simulink model "BatterySimulation"  (R2024a)
settings: Solver=VariableStepAuto  StartTime=0.0  StopTime=inf  FixedStep=minStep  MaxStep=(1e-5)*1000  MinStep=1e-5  RelTol=1e-3
libraries: fl_lib x7, nesl_utility x4, batteryecm_lib x1, simulink x1
settings Model: SimulationMode=accelerator  Creator=nsu  LastModifiedBy=nsu

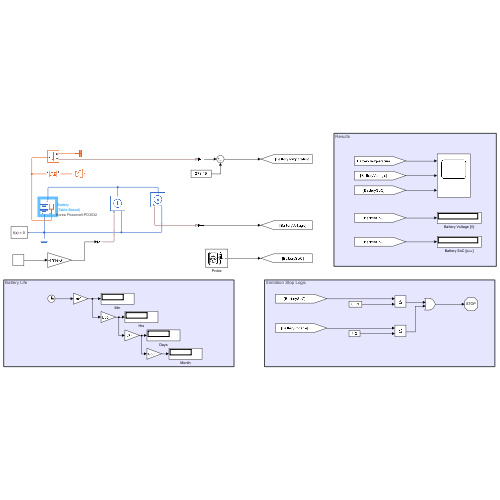
[thumbnail: Simulink's stored preview of the top-level diagram]
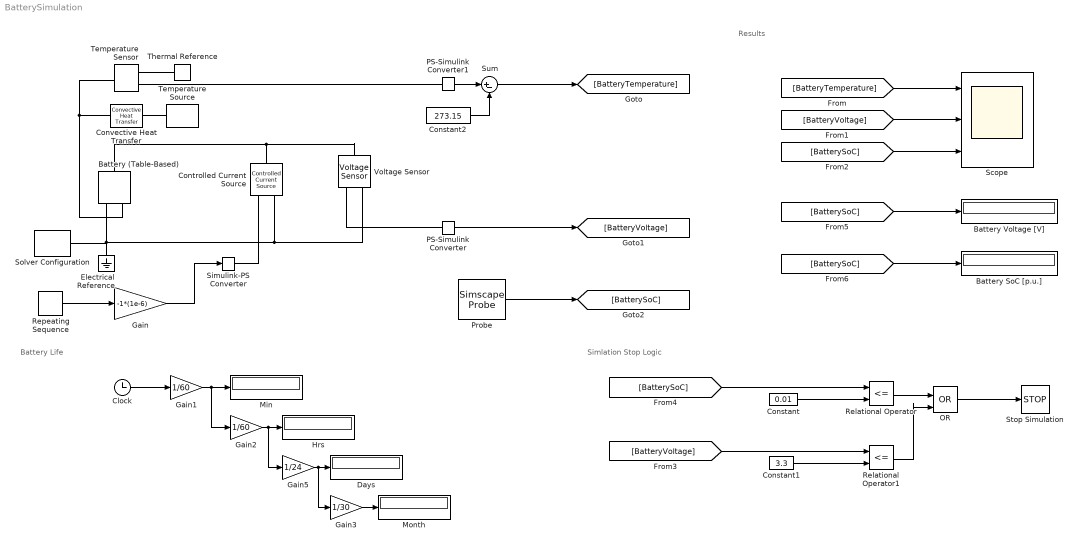
== system BatterySimulation ==
  note: Results
  note: Simlation Stop Logic
  note: Battery Life
  Battery (Table-Based) : batteryecm_lib/Battery (Table-Based)  Tag={'toolbox/physmod/battery/shared_library/m/batteryecm_lib_parts';'Battery__Table_Based_/Korea_Powercell/PD3032.xml'}  SOC_vec=[0 0.01 0.02 0.03 0.04 0.05 0.06 0.07 0.08 0.09 0.1 0.11 0.12 0.13 0.14 0.15 0.16 0.17 0.18 0.19 0.2 0.21 0.22 0.23 0.24 0.25 0.26 0.27 0.28 0.29 0.3 0.31 0.32 0.33 0.34 0.35 0.36 0.37 0.38 0.39 0.4 0.41 0.42 0.43 0.44 0.45 0.46 0.47 0.48 0.49 0.5 0.51 0.52 0.53 0.54 0.55 0.56 0.57 0.58 0.59 0.6 0.61 0.62 0.63 0.64 0.65 0.66 0.67 0.68 0.69 0.7 0.71 0.72 0.73 0.74 0.75 0.76 0.77 0.78 0.79 0.8 0.81 0.82 0.83 0.84 0.85 0.86 0.87 0.88 0.89 0.9 0.91 0.92 0.93 0.94 0.95 0.96 0.97 0.98 0.99 1]  T_dependence=simscape.enum.tablebattery.temperature_dependence.yes  prm_dir=simscape.enum.tablebattery.prm_dir.noCurrentDirectionality  T_vec=[-20 -10 25] degC  V0_mat=[2.95724 2.95724 2.95724;3.3564 3.3564 3.3564;3.49366 3.49366 3.49366;3.58258 3.58258 3.58258;3.63766 3.63766 3.63766;3.68332 3.68332 3.68332;3.70873 3.70873 3.70873;3.73055 3.73055 3.73055;3.74166 3.74166 3.74166;3.74045 3.74045 3.74045;3.73776 3.73776 3.73776;3.73631 3.73631 3.73631;3.73521 3.73521 3.73521;3.73661 3.73661 3.73661;3.73787 3.73787 3.73787;3.73862 3.73862 3.73862;3.74076 3.74076 3.74076;3.74303 3.74303 3.74303;3.74502 3.74502 3.74502;3.7472 3.7472 3.7472;3.74981 3.74981 3.74981;3.75229 3.75229 3.75229;3.7538 3.7538 3.7538;3.75584 3.75584 3.75584;3.75779 3.75779 3.75779;3.75969 3.75969 3.75969;3.76148 3.76148 3.76148;3.76318 3.76318 3.76318;3.76489 3.76489 3.76489;3.76695 3.76695 3.76695;3.76868 3.76868 3.76868;3.77025 3.77025 3.77025;3.77183 3.77183 3.77183;3.77343 3.77343 3.77343;3.77506 3.77506 3.77506;3.77658 3.77658 3.77658;3.77841 3.77841 3.77841;3.78029 3.78029 3.78029;3.78217 3.78217 3.78217;3.78415 3.78415 3.78415;3.78659 3.78659 3.78659;3.78921 3.78921 3.78921;3.79241 3.79241 3.79241;3.7956 3.7956 3.7956;3.79881 3.79881 3.79881;3.80207 3.80207 3.80207;3.80534 3.80534 3.80534;3.80863 3.80863 3.80863;3.81212 3.81212 3.81212;3.81572 3.81572 3.81572;3.81951 3.81951 3.81951;3.8234 3.8234 3.8234;3.82746 3.82746 3.82746;3.83153 3.83153 3.83153;3.83559 3.83559 3.83559;3.83995 3.83995 3.83995;3.8442 3.8442 3.8442;3.84844 3.84844 3.84844;3.85268 3.85268 3.85268;3.85692 3.85692 3.85692;3.86126 3.86126 3.86126;3.86664 3.86664 3.86664;3.87235 3.87235 3.87235;3.87807 3.87807 3.87807;3.8838 3.8838 3.8838;3.88953 3.88953 3.88953;3.89582 3.89582 3.89582;3.90255 3.90255 3.90255;3.90959 3.90959 3.90959;3.91623 3.91623 3.91623;3.92281 3.92281 3.92281;3.92954 3.92954 3.92954;3.93614 3.93614 3.93614;3.94227 3.94227 3.94227;3.94795 3.94795 3.94795;3.9535 3.9535 3.9535;3.9591 3.9591 3.9591;3.96511 3.96511 3.96511;3.97114 3.97114 3.97114;3.97777 3.97777 3.97777;3.98488 3.98488 3.98488;3.99222 3.99222 3.99222;4.00167 4.00167 4.00167;4.01113 4.01113 4.01113;4.02255 4.02255 4.02255;4.03398 4.03398 4.03398;4.04484 4.04484 4.04484;4.05571 4.05571 4.05571;4.06578 4.06578 4.06578;4.07395 4.07395 4.07395;4.08139 4.08139 4.08139;4.08919 4.08919 4.08919;4.09698 4.09698 4.09698;4.10586 4.10586 4.10586;4.11561 4.11561 4.11561;4.12482 4.12482 4.12482;4.13514 4.13514 4.13514;4.1452 4.1452 4.1452;4.15846 4.15846 4.15846;4.17552 4.17552 4.17552;4.19579 4.19579 4.19579] V  V0_vec=[2.95724 3.3564 3.49366 3.58258 3.63766 3.68332 3.70873 3.73055 3.74166 3.74045 3.73776 3.73631 3.73521 3.73661 3.73787 3.73862 3.74076 3.74303 3.74502 3.7472 3.74981 3.75229 3.7538 3.75584 3.75779 3.75969 3.76148 3.76318 3.76489 3.76695 3.76868 3.77025 3.77183 3.77343 3.77506 3.77658 3.77841 3.78029 3.78217 3.78415 3.78659 3.78921 3.79241 3.7956 3.79881 3.80207 3.80534 3.80863 3.81212 3.81572 3.81951 3.8234 3.82746 3.83153 3.83559 3.83995 3.8442 3.84844 3.85268 3.85692 3.86126 3.86664 3.87235 3.87807 3.8838 3.88953 3.89582 3.90255 3.90959 3.91623 3.92281 3.92954 3.93614 3.94227 3.94795 3.9535 3.9591 3.96511 3.97114 3.97777 3.98488 3.99222 4.00167 4.01113 4.02255 4.03398 4.04484 4.05571 4.06578 4.07395 4.08139 4.08919 4.09698 4.10586 4.11561 4.12482 4.13514 4.1452 4.15846 4.17552 4.19579] V  V_range=[2.475 Inf] V  R0_mat=[13.06476 14.44423 0.86823;29.81327 21.8324 1.97565;29.32491 20.9161 2.19839;28.83655 19.9998 2.30336;28.34819 18.19935 2.32493;27.85984 17.50082 2.32311;27.37148 16.61595 2.27325;26.88312 15.89183 2.21593;26.09738 14.90922 2.13322;25.03793 13.65137 2.00795;24.00131 12.81743 1.88032;23.00792 12.0179 1.79212;22.19973 11.22784 1.70777;21.46135 10.62953 1.65332;20.7188 10.03863 1.59953;20.00887 9.43363 1.54628;19.42784 9.00253 1.51052;18.85043 8.62654 1.47625;18.26513 8.24266 1.44119;17.68531 7.86426 1.41044;17.13317 7.58083 1.38852;16.6795 7.35612 1.36656;16.19909 7.10467 1.34119;15.73321 6.93534 1.32173;15.27136 6.76528 1.30512;14.88815 6.59399 1.28839;14.50155 6.41932 1.27179;14.11281 6.24252 1.25526;13.72408 6.06571 1.23874;13.34509 5.899 1.2262;13.02865 5.80696 1.21367;12.71874 5.71056 1.20059;12.40882 5.61416 1.1875;12.09982 5.51868 1.17438;11.79134 5.42372 1.1611;11.50108 5.3259 1.14754;11.26645 5.23787 1.13738;11.03344 5.1536 1.12789;10.80043 5.06933 1.11839;10.57531 4.98781 1.10879;10.42886 4.91904 1.10081;10.28743 4.85528 1.09337;10.16188 4.8185 1.08812;10.03643 4.81547 1.08292;9.91124 4.81269 1.0777;9.78779 4.81165 1.07242;9.66434 4.81062 1.06713;9.54138 4.81007 1.0619;9.42854 4.81539 1.0576;9.34107 4.81015 1.05404;9.25891 4.79214 1.05115;9.17945 4.77683 1.04816;9.10496 4.76649 1.04499;9.03048 4.75616 1.04181;8.95599 4.74582 1.03864;8.88964 4.74362 1.03566;8.82825 4.73821 1.0296;8.77948 4.7379 1.02355;8.73072 4.73595 1.0175;8.68196 4.72311 1.01145;8.6359 4.71298 1.00529;8.61851 4.73151 1.00231;8.61048 4.74855 1.00071;8.58703 4.74062 0.99934;8.5589 4.73268 0.99797;8.53075 4.72471 0.99661;8.51821 4.73235 0.997;8.51779 4.7536 0.99877;8.52615 4.78798 1.00166;8.52341 4.81126 1.00003;8.53059 4.83287 0.9977;8.5517 4.85841 0.99522;8.5693 4.88044 0.99239;8.57397 4.8921 0.98804;8.56628 4.89917 0.97908;8.55463 4.90228 0.96851;8.53748 4.90689 0.95788;8.50069 4.92307 0.94772;8.4643 4.93965 0.9376;8.44446 4.97278 0.93052;8.43829 4.99602 0.92549;8.43805 4.96358 0.92024;8.48079 4.99015 0.91984;8.48047 5.01696 0.91946;8.53436 5.09799 0.92519;8.5886 5.16658 0.93088;8.62702 5.08225 0.93501;8.6658 4.99828 0.93884;8.62871 4.89202 0.93969;8.49214 4.73309 0.93315;8.33515 4.55373 0.91826;8.18823 4.40985 0.90491;7.99248 4.30829 0.89156;7.8008 4.23692 0.88207;7.6331 4.18953 0.87038;7.45051 4.12724 0.84466;7.2987 4.06626 0.81895;7.04671 3.86682 0.79033;6.71527 3.75645 0.74611;6.48896 3.75121 0.69824;4.40131 2.41048 0.5801] Ohm  R0_vec=[0.86823 1.97565 2.19839 2.30336 2.32493 2.32311 2.27325 2.21593 2.13322 2.00795 1.88032 1.79212 1.70777 1.65332 1.59953 1.54628 1.51052 1.47625 1.44119 1.41044 1.38852 1.36656 1.34119 1.32173 1.30512 1.28839 1.27179 1.25526 1.23874 1.2262 1.21367 1.20059 1.1875 1.17438 1.1611 1.14754 1.13738 1.12789 1.11839 1.10879 1.10081 1.09337 1.08812 1.08292 1.0777 1.07242 1.06713 1.0619 1.0576 1.05404 1.05115 1.04816 1.04499 1.04181 1.03864 1.03566 1.0296 1.02355 1.0175 1.01145 1.00529 1.00231 1.00071 0.99934 0.99797 0.99661 0.997 0.99877 1.00166 1.00003 0.9977 0.99522 0.99239 0.98804 0.97908 0.96851 0.95788 0.94772 0.9376 0.93052 0.92549 0.92024 0.91984 0.91946 0.92519 0.93088 0.93501 0.93884 0.93969 0.93315 0.91826 0.90491 0.89156 0.88207 0.87038 0.84466 0.81895 0.79033 0.74611 0.69824 0.5801] Ohm  R0_dis_mat=[.0117, .0085, .009; .011, .0085, .009; .0114, .0087, .0092; .0107, .0082, .0088; .0107, .0083, .0091; .0113, .0085, .0089; .0116, .0085, .0089] % Parameter not set Ohm  R0_dis_vec=[.0085, .0085, .0087, .0082, .0083, .0085, .0085] % Parameter not set Ohm  R0_ch_mat=[.0117, .0085, .009; .011, .0085, .009; .0114, .0087, .0092; .0107, .0082, .0088; .0107, .0083, .0091; .0113, .0085, .0089; .0116, .0085, .0089] % Parameter not set Ohm  R0_ch_vec=[.0085, .0085, .0087, .0082, .0083, .0085, .0085] % Parameter not set Ohm  AH=0.192 hr*A  prm_leak=simscape.enum.tablebattery.prm_leak.disabled  Rleak_vec=[8000, 7000, 6000] % Parameter not set Ohm  Rleak=7e3 % Parameter not set Ohm  extrapolation_option=simscape.enum.extrapolation.nearest  SOC_port=simscape.enum.tablebattery.enable.no  prm_dyn=simscape.enum.tablebattery.prm_dyn.off  R1_mat=[.0109, .0029, .0013; .0069, .0024, .0012; .0047, .0026, .0013; .0034, .0016, .001; .0033, .0023, .0014; .0033, .0018, .0011; .0028, .0017, .0011] % Parameter not set Ohm  R1_vec=[.0029, .0024, .0026, .0016, .0023, .0018, .0017] % Parameter not set Ohm  tau1_mat=[20, 36, 39; 31, 45, 39; 109, 105, 61; 36, 29, 26; 59, 77, 67; 40, 33, 29; 25, 39, 33] % Parameter not set s  tau1_vec=[36, 45, 105, 29, 77, 33, 39] % Parameter not set s  R2_mat=[.0109, .0029, .0013; .0069, .0024, .0012; .0047, .0026, .0013; .0034, .0016, .001; .0033, .0023, .0014; .0033, .0018, .0011; .0028, .0017, .0011] % Parameter not set Ohm  R2_vec=[.0029, .0024, .0026, .0016, .0023, .0018, .0017] % Parameter not set Ohm  tau2_mat=[20, 36, 39; 31, 45, 39; 109, 105, 61; 36, 29, 26; 59, 77, 67; 40, 33, 29; 25, 39, 33] % Parameter not set s  tau2_vec=[36, 45, 105, 29, 77, 33, 39] % Parameter not set s  R3_mat=[.0109, .0029, .0013; .0069, .0024, .0012; .0047, .0026, .0013; .0034, .0016, .001; .0033, .0023, .0014; .0033, .0018, .0011; .0028, .0017, .0011] % Parameter not set Ohm  R3_vec=[.0029, .0024, .0026, .0016, .0023, .0018, .0017] % Parameter not set Ohm  tau3_mat=[20, 36, 39; 31, 45, 39; 109, 105, 61; 36, 29, 26; 59, 77, 67; 40, 33, 29; 25, 39, 33] % Parameter not set s  tau3_vec=[36, 45, 105, 29, 77, 33, 39] % Parameter not set s  R4_mat=[.0109, .0029, .0013; .0069, .0024, .0012; .0047, .0026, .0013; .0034, .0016, .001; .0033, .0023, .0014; .0033, .0018, .0011; .0028, .0017, .0011] % Parameter not set Ohm  R4_vec=[.0029, .0024, .0026, .0016, .0023, .0018, .0017] % Parameter not set Ohm  tau4_mat=[20, 36, 39; 31, 45, 39; 109, 105, 61; 36, 29, 26; 59, 77, 67; 40, 33, 29; 25, 39, 33] % Parameter not set s  tau4_vec=[36, 45, 105, 29, 77, 33, 39] % Parameter not set s  R5_mat=[.0109, .0029, .0013; .0069, .0024, .0012; .0047, .0026, .0013; .0034, .0016, .001; .0033, .0023, .0014; .0033, .0018, .0011; .0028, .0017, .0011] % Parameter not set Ohm  R5_vec=[.0029, .0024, .0026, .0016, .0023, .0018, .0017] % Parameter not set Ohm  tau5_mat=[20, 36, 39; 31, 45, 39; 109, 105, 61; 36, 29, 26; 59, 77, 67; 40, 33, 29; 25, 39, 33] % Parameter not set s  tau5_vec=[36, 45, 105, 29, 77, 33, 39] % Parameter not set s  prm_fade=simscape.enum.tablebattery.prm_fade.tableN  N0=100 % Parameter not set  dV0=0 % Parameter not set  dR0=0 % Parameter not set  dAH=0 % Parameter not set  dRleak=0 % Parameter not set  dR1=0 % Parameter not set  dR2=0 % Parameter not set  dR3=0 % Parameter not set  dR4=0 % Parameter not set  dR5=0 % Parameter not set  N0vec=[0 7 13 19 25 31 37 43 49 55 61 67 73 79 85 91 97 103 109 115 121 127 133 139 145 151 157 163 169 175 181 187 193 199 205 211 217 223 229 235 241 247 253 259 265 271 277 283 289 295 301 307 313 319 325 331 337 343 349 355 361 367 373 379 385 391 397 403 409 415 421 427 433 439 445 451 457 463 469 475 481 487 493 499]  Tfadevec=[298.15, 323.15] % Parameter not set K  dV0vec=[0 -0.0628 -0.1257 -0.1885 -0.2514 -0.3142 -0.3771 -0.4515 -0.562 -0.6675 -0.7729 -0.8784 -0.9629 -1.0447 -1.1233 -1.202 -1.2626 -1.3222 -1.3819 -1.4415 -1.5026 -1.5637 -1.6249 -1.6861 -1.7412 -1.7958 -1.8504 -1.905 -1.9604 -2.0097 -2.059 -2.1083 -2.1563 -2.2012 -2.2461 -2.291 -2.3359 -2.3776 -2.4217 -2.4669 -2.5121 -2.5574 -2.6026 -2.6479 -2.6931 -2.7378 -2.7708 -2.8037 -2.8367 -2.8696 -2.9026 -2.9386 -2.9748 -3.011 -3.0472 -3.0834 -3.1244 -3.1642 -3.2017 -3.2391 -3.2765 -3.3139 -3.3524 -3.3928 -3.4325 -3.4721 -3.5117 -3.5513 -3.5909 -3.6304 -3.67 -3.7095 -3.7605 -3.8167 -3.8738 -3.9329 -3.992 -4.0512 -4.1103 -4.1478 -4.1826 -4.2174 -4.2523 -4.2871]  dR0vec=[0 0 0 0 0 0 0 0 0 0 0 0 0 0 0 0 0 0 0 0 0 0 0 0 0 0 0 0 0 0 0 0 0 0 0 0 0 0 0 0 0 0 0 0 0 0 0 0 0 0 0 0 0 0 0 0 0 0 0 0 0 0 0 0 0 0 0 0 0 0 0 0 0 0 0 0 0 0 0 0 0 0 0 0] % Parameter assumed  dAHvec=[0 -0.13 -0.26 -0.39 -0.52 -0.65 -0.78 -0.934 -1.194 -1.453 -1.713 -1.972 -2.232 -2.49 -2.739 -2.988 -3.236 -3.485 -3.734 -3.983 -4.231 -4.48 -4.729 -4.978 -5.226 -5.475 -5.724 -5.973 -6.213 -6.425 -6.637 -6.849 -7.061 -7.273 -7.486 -7.698 -7.91 -8.122 -8.359 -8.602 -8.846 -9.089 -9.333 -9.576 -9.82 -10.063 -10.249 -10.435 -10.621 -10.806 -10.992 -11.178 -11.364 -11.55 -11.736 -11.921 -12.107 -12.273 -12.429 -12.585 -12.741 -12.897 -13.053 -13.209 -13.362 -13.515 -13.668 -13.82 -13.973 -14.126 -14.279 -14.432 -14.629 -14.846 -15.063 -15.28 -15.497 -15.714 -15.932 -16.069 -16.197 -16.325 -16.453 -16.581]  dRleakvec=[0, 0, 0, 0] % Parameter not set  dR1vec=[0, 0, 0, 0] % Parameter not set  dR2vec=[0, 0, 0, 0] % Parameter not set  dR3vec=[0, 0, 0, 0] % Parameter not set  dR4vec=[0, 0, 0, 0] % Parameter not set  dR5vec=[0, 0, 0, 0] % Parameter not set  dV0mat=[0, 0; 0, 0; 0, 0; 0, 0] % Parameter not set  dR0mat=[0, 0; 0, 0; 0, 0; 0, 0] % Parameter not set  dAHmat=[0, 0; 0, 0; 0, 0; 0, 0] % Parameter not set  dRleakmat=[0, 0; 0, 0; 0, 0; 0, 0] % Parameter not set  dR1mat=[0, 0; 0, 0; 0, 0; 0, 0] % Parameter not set  dR2mat=[0, 0; 0, 0; 0, 0; 0, 0] % Parameter not set  dR3mat=[0, 0; 0, 0; 0, 0; 0, 0] % Parameter not set  dR4mat=[0, 0; 0, 0; 0, 0; 0, 0] % Parameter not set  dR5mat=[0, 0; 0, 0; 0, 0; 0, 0] % Parameter not set  prm_age_modeling=simscape.enum.tablebattery.prm_age_modeling.equation  storage_dt_age_vec=[0] % Parameter not set d  storage_T_age_vec=[273] % Parameter not set K  prm_age_OCV=simscape.enum.tablebattery.prm_age_OCV.OCV  OCV_age=0.9 % Parameter not set  SOC_age=0.6 % Parameter not set  prm_age_resistance=simscape.enum.tablebattery.prm_age.disabled  OCV_scaling_age_resistance=2.2134e6 % Parameter not set  OCV_offset_age_resistance=1.632e6 % Parameter not set  temp_exp_age_resistance=0.515833569 % Parameter not set V  t_exp_age_resistance=0.75 % Parameter not set  T_age_vec_resistance=[273.15, 298.15, 323.15] % Parameter not set K  dt_age_vec_resistance=[0, 90, 180, 270] % Parameter not set d  dR0_age_vec=[0, 0, 0] % Parameter not set  t_meas_dR0_age=100 % Parameter not set d  dR0_age_mat=[0, 0, 0; 0, 0, 0; 0, 0, 0; 0, 0, 0] % Parameter not set  prm_age_capacity=simscape.enum.tablebattery.prm_age.disabled  OCV_scaling_age_capacity=1.5097e07 % Parameter not set  OCV_offset_age_capacity=8.3625e06 % Parameter not set  temp_exp_age_capacity=0.6011 % Parameter not set V  t_exp_age_capacity=0.75 % Parameter not set  T_age_vec_capacity=[273.15, 298.15, 323.15] % Parameter not set K  dt_age_vec_capacity=[0, 90, 180, 270] % Parameter not set d  dAH_age_vec=[0, 0, 0] % Parameter not set  t_meas_dAH_age=100 % Parameter not set d  dAH_age_mat=[0, 0, 0; 0, 0, 0; 0, 0, 0; 0, 0, 0] % Parameter not set  thermal_port=simscape.enum.thermaleffects.model  temperature=298.15 % Parameter not set K  thermal_mass=6.48 % Parameter assumed J/K  i_specify=off  i_priority=None  i=0 A  i_nominal_specify=off  i_nominal_value=1  i_nominal_unit=A  v_specify=off  v_priority=None  v=0 V  v_nominal_specify=off  v_nominal_value=1  v_nominal_unit=V  stateOfCharge_specify=off  stateOfCharge_priority=High  stateOfCharge=1  stateOfCharge_nominal_specify=off  stateOfCharge_nominal_value=1  stateOfCharge_nominal_unit=1  num_cycles_specify=off  num_cycles_priority=High  num_cycles=0  num_cycles_nominal_specify=off  num_cycles_nominal_value=1  num_cycles_nominal_unit=1  cell_temperature_specify=off  cell_temperature_priority=High  cell_temperature=298.15 K  cell_temperature_nominal_specify=off  cell_temperature_nominal_value=1  cell_temperature_nominal_unit=K
      settings: AttributesFormatString=Korea Powercell:PD3032  InternalSimscapePortConfiguration="{\"Bottom\":[],\"Left\":[{\"id\":\"p\",\"label\":\"+\",\"type\":\"foundation.electrical.electrical\"}],\"Right\":[{\"id\":\"n\",\"label\":\"-\",\"type\":\"foundation.electrical.electrical\"},{\"id\":\"H\",\"label\":\"H\",\"type\":\"foundation.thermal.thermal\"}],\"Top\":[]}"
      settings: LibrarySourceBlock=|
      | batt_lib/Cells/Battery
      | (Table-Based)
  Battery SoC [p.u.] : Display
      settings: Decimation=100
  Battery Voltage [V] : Display
      settings: Decimation=100
  Clock : Clock
  Constant : Constant  Value=0.01
  Constant1 : Constant  Value=3.3
  Constant2 : Constant  Value=273.15
  Controlled Current Source : fl_lib/Electrical/Electrical Sources/Controlled Current Source
  Convective Heat Transfer : fl_lib/Thermal/Thermal Elements/Convective Heat Transfer  thermal_type=foundation.enum.constant_variable.constant  area=1e-4 m^2  heat_tr_coeff=20 W/(K*m^2)  min_heat_tr_coeff=1e-3 W/(K*m^2)  T_specify=off  T_priority=None  T=0 K  T_nominal_specify=off  T_nominal_value=1  T_nominal_unit=K  Q_specify=off  Q_priority=None  Q=0 W  Q_nominal_specify=off  Q_nominal_value=1  Q_nominal_unit=W
  Days : Display
      settings: Decimation=100
  Electrical Reference : fl_lib/Electrical/Electrical Elements/Electrical Reference
  Gain : Gain  Gain=-1*(1e-6)
  Gain1 : Gain  Gain=1/60
  Gain2 : Gain  Gain=1/60
  Gain3 : Gain  Gain=1/30
  Gain5 : Gain  Gain=1/24
  Hrs : Display
      settings: Decimation=100
  Min : Display
      settings: Decimation=100
  Month : Display
      settings: Decimation=100
  OR : Logic  Operator=OR  IconShape=distinctive  AllPortsSameDT=off  OutDataTypeStr=boolean
  PS-Simulink Converter : nesl_utility/PS-Simulink Converter  PhysicalDomain=network_engine_domain  SubClassName=ps_output  LeftPortType=input  RightPortType=output  PseudoPeriodic=off  Frequencies=[]  VectorFormat=inherit  Unit=inherit  AffineConversion=off
  PS-Simulink Converter1 : nesl_utility/PS-Simulink Converter  PhysicalDomain=network_engine_domain  SubClassName=ps_output  LeftPortType=input  RightPortType=output  PseudoPeriodic=off  Frequencies=[]  VectorFormat=inherit  Unit=inherit  AffineConversion=off
  Probe : SimscapeProbe  BoundBlock=12  Variables={stateOfCharge}
  Relational Operator : RelationalOperator  Operator=<=  OutDataTypeStr=boolean  RndMeth=Simplest  InputSameDT=off
  Relational Operator1 : RelationalOperator  Operator=<=  OutDataTypeStr=boolean  RndMeth=Simplest  InputSameDT=off
  Repeating Sequence : simulink/Sources/Repeating Sequence  rep_seq_t=time  rep_seq_y=current
  Scope : Scope  NumInputPorts=3
  Simulink-PS Converter : nesl_utility/Simulink-PS Converter  PhysicalDomain=network_engine_domain  SubClassName=ps_input  LeftPortType=input  RightPortType=output  PseudoPeriodic=off  Frequencies=[]  NoiseDistribution=none  NoiseParameters=[]  Unit=1  AffineConversion=off  FilteringAndDerivatives=provide  SimscapeFilterOrder=1  InputFilterTimeConstant=0.001  UdotUserProvided=0
  Solver Configuration : nesl_utility/Solver Configuration  PhysicalDomain=network_engine_domain  SubClassName=solver  LeftPortType=input  RightPortType=generic  Tones=[]  Harmonics=[]  SimulateNoise=off  Profile=off  UseLocalSampling=off  EnableSwitchedLinearOptims=on  FrequencyDomain=off  UseCCode=off  RelTol=0.001  AbsTol=0.001  MinStep=1e-09  ToWorkspace=off  RevertToSquareIcSolve=off  NumHomotopyIterations=100  PhasorMode=off  PhasorModeNumHarmonics=1  ConsistencySolver=NEWTON_XTOL_AFTER_FTOL  IndexReductionMethod=DerivativeReplacement  DoDC=off  ResidualTolerance=1e-09  ConsistencyTolSource=GLOBAL  ConsistencyAbsTol=0.001  ConsistencyRelTol=0.001  ConsistencyTolFactor=0.001  UseLocalSolver=off  LocalSolverChoice=NE_BACKWARD_EULER_ADVANCER  ResolveIndetEquations=on  FunctionEvalNumThread=1  LocalSolverSampleTime=0.01  DoFixedCost=off  MaxNonlinIter=3  MaxModeIter=2  ComputeImpulses=off  ImpulseIterations=2  LinearAlgebra=auto  LinearAlgebraNumThread=0  EquationFormulation=NE_TIME_EF  DelaysMemoryBudget=1024  AutomaticFiltering=on  FilteringTimeConstant=0.001  PartitionStorageMethod=AS_NEEDED  PartitionMemoryBudget=1024  PartitionMethod=ROBUST  MultibodyUseLocalSolver=off  MultibodyLocalSolverChoice=ODE1  MultibodyLocalSolverSampleTime=0.001
  Stop Simulation : Stop
  Sum : Sum  Inputs=|+-
  Temperature Sensor : fl_lib/Thermal/Thermal Sensors/Temperature Sensor  temperature_measure=foundation.enum.MeasurementReference.difference
  Temperature Source : fl_lib/Thermal/Thermal Sources/Temperature Source  temperature=310.15 K
  Thermal Reference : fl_lib/Thermal/Thermal Elements/Thermal Reference
  Voltage Sensor : fl_lib/Electrical/Electrical Sensors/Voltage Sensor
  wires:
  Gain/1 -> Simulink-PS Converter/1
  Repeating Sequence/1 -> Gain/1
  Constant/1 -> Relational Operator/2
  Clock/1 -> Gain1/1
  Gain1/1 -> Gain2/1, Min/1
  Gain2/1 -> Gain5/1, Hrs/1
  Gain5/1 -> Gain3/1, Days/1
  Gain3/1 -> Month/1
  Constant1/1 -> Relational Operator1/2
  Relational Operator/1 -> OR/1
  Relational Operator1/1 -> OR/2
  OR/1 -> Stop Simulation/1
  PS-Simulink Converter1/1 -> Sum/1
  Constant2/1 -> Sum/2
  Sum/1 -> [BatteryTemperature]
  [BatteryTemperature] -> Scope/1
  PS-Simulink Converter/1 -> [BatteryVoltage]
  [BatteryVoltage] -> Scope/2
  Probe/1 -> [BatterySoC]
  [BatterySoC] -> Scope/3
  [BatteryVoltage] -> Relational Operator1/1
  [BatterySoC] -> Relational Operator/1
  [BatterySoC] -> Battery Voltage [V]/1
  [BatterySoC] -> Battery SoC [p.u.]/1
  connections:
  Battery (Table-Based)/LConn1 -- Voltage Sensor/LConn1 -- Controlled Current Source/LConn1
  Battery (Table-Based)/RConn1 -- Solver Configuration/RConn1 -- Electrical Reference/LConn1 -- Voltage Sensor/RConn2 -- Controlled Current Source/RConn2
  Simulink-PS Converter/RConn1 -- Controlled Current Source/RConn1
  PS-Simulink Converter/LConn1 -- Voltage Sensor/RConn1
  Temperature Sensor/LConn1 -- Convective Heat Transfer/LConn1 -- Battery (Table-Based)/RConn2
  Temperature Source/LConn1 -- Convective Heat Transfer/RConn1
  Temperature Sensor/RConn2 -- PS-Simulink Converter1/LConn1
  Thermal Reference/LConn1 -- Temperature Sensor/RConn1
